simulink model "detumbling"  (R2021a)
settings: Solver=VariableStepAuto  StartTime=0.0  StopTime=3*Torb  RelTol=1e-3
values from neighbouring files (symbols this model uses):
  inc = 0    [params_detumb.m]    (also in params_nadir.m; params_roll.m)
  Torb = 2*pi*sqrt(norm(r0)^3/mu)    [params_detumb.m]    (also in params_nadir.m; params_roll.m)
libraries: sharedtransform x5, aerolibutil x2
settings Model: Creator=Laura  LastModifiedBy=Laura

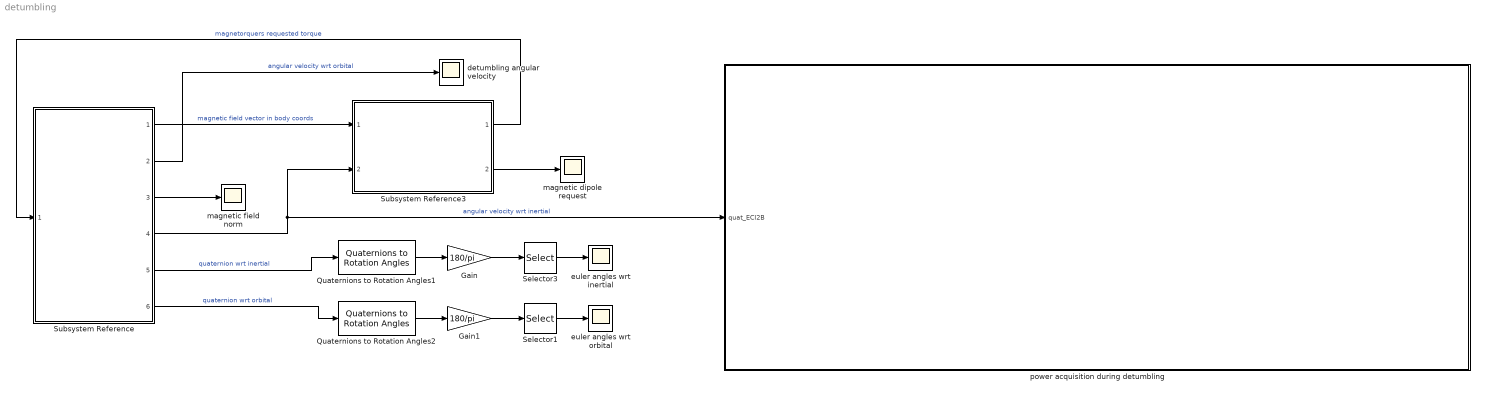
== system detumbling ==
  Gain : Gain  Gain=180/pi
  Gain1 : Gain  Gain=180/pi
  Quaternions to Rotation Angles1 : sharedtransform/Quaternions to Rotation Angles  rotationOrder=ZYX  aMode=aMode
      settings: SourceProductBaseCode=AE,PW,DR,MT,UV,VE
  Quaternions to Rotation Angles2 : sharedtransform/Quaternions to Rotation Angles  rotationOrder=ZYX  aMode=aMode
      settings: SourceProductBaseCode=AE,PW,DR,MT,UV,VE
  Selector1 : Selector  InputPortWidth=3  IndexOptions=Index vector (dialog)  Indices=[3 2 1]  OutputSizes=1
  Selector3 : Selector  InputPortWidth=3  IndexOptions=Index vector (dialog)  Indices=[3 2 1]  OutputSizes=1
  Subsystem Reference : Subsystem  ReferencedSubsystem=DKE
  Subsystem Reference3 : Subsystem  ReferencedSubsystem=BdotController
  detumbling angular velocity : Scope
  euler angles wrt inertial : Scope
  euler angles wrt orbital : Scope
  magnetic dipole request : Scope
  magnetic field norm : Scope
  power acquisition during detumbling : Subsystem
  wires:
  Quaternions to Rotation Angles1/1 -> Gain/1
  Gain/1 -> Selector3/1
  Selector3/1 -> euler angles wrt inertial/1
  Subsystem Reference/1 -> Subsystem Reference3/1  "magnetic field vector in body coords"
  Subsystem Reference/2 -> detumbling angular velocity/1  "angular velocity wrt orbital"
  Subsystem Reference3/1 -> Subsystem Reference/1  "magnetorquers requested torque"
  Quaternions to Rotation Angles2/1 -> Gain1/1
  Subsystem Reference/4 -> power acquisition during detumbling/1(quat_ECI2B), Subsystem Reference3/2  "angular velocity wrt inertial"
  Subsystem Reference/3 -> magnetic field norm/1
  Gain1/1 -> Selector1/1
  Selector1/1 -> euler angles wrt orbital/1
  Subsystem Reference/6 -> Quaternions to Rotation Angles2/1  "quaternion wrt orbital"
  Subsystem Reference/5 -> Quaternions to Rotation Angles1/1  "quaternion wrt inertial"
  Subsystem Reference3/2 -> magnetic dipole request/1

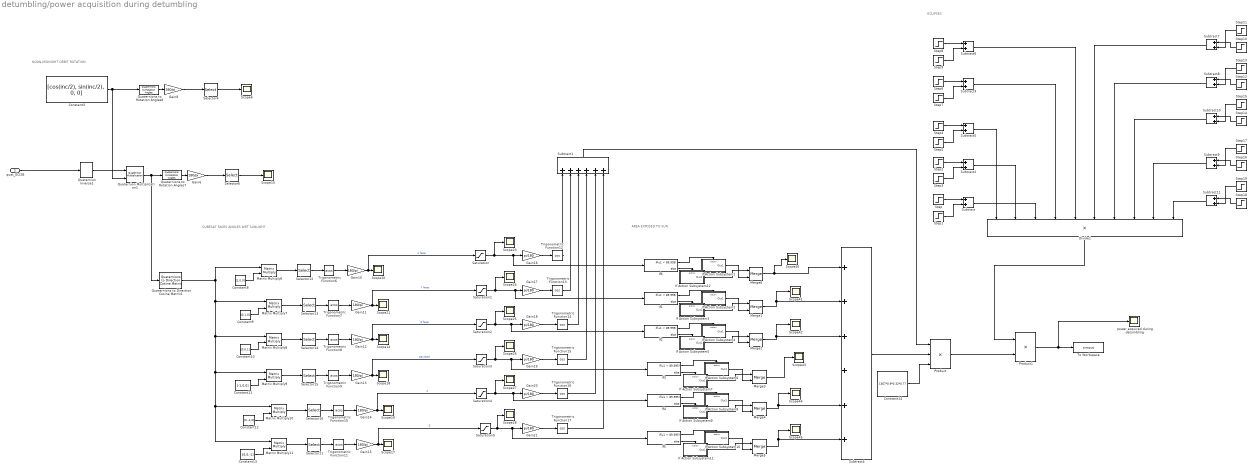
== system detumbling/power acquisition during detumbling ==
  note: AREA EXPOSED TO SUN
  note: ECLIPSES
  note: CUBESAT FACES ANGLES WRT SUNLIGHT
  note: NOON-MIDNIGHT ORBIT ROTATION
  quat_ECI2B : Inport
  Constant10 : Constant  Value=[0,0,1]
  Constant11 : Constant  Value=[-1,0,0]
  Constant12 : Constant  Value=[0,-1,0]
  Constant13 : Constant  Value=[0,0,-1]
  Constant14 : Constant  Value=1367*0.9*0.32*0.77
  Constant3 : Constant  Value=[cos(inc/2), sin(inc/2), 0, 0]
  Constant8 : Constant  Value=[1,0,0]
  Constant9 : Constant  Value=[0,1,0]
  Divide1 : Product  Inputs=**********
  Gain{6,8,10..15} (8 alike) : Gain  Gain=180/pi
  Gain{16..21} (6 alike) : Gain  Gain=pi/180
  If Action Subsystem1 : Subsystem  TreatAsAtomicUnit=on
  If Action Subsystem10 : Subsystem  TreatAsAtomicUnit=on
  If Action Subsystem11 : Subsystem  TreatAsAtomicUnit=on
  If Action Subsystem12 : Subsystem  TreatAsAtomicUnit=on
  If Action Subsystem2 : Subsystem  TreatAsAtomicUnit=on
  If Action Subsystem3 : Subsystem  TreatAsAtomicUnit=on
  If Action Subsystem4 : Subsystem  TreatAsAtomicUnit=on
  If Action Subsystem5 : Subsystem  TreatAsAtomicUnit=on
  If Action Subsystem6 : Subsystem  TreatAsAtomicUnit=on
  If Action Subsystem7 : Subsystem  TreatAsAtomicUnit=on
  If Action Subsystem8 : Subsystem  TreatAsAtomicUnit=on
  If Action Subsystem9 : Subsystem  TreatAsAtomicUnit=on
  If{1..6} (6 alike) : If  IfExpression=u1 < 89.995
  Matrix Multiply{6..11} (6 alike) : Product  Multiplication=Matrix(*)
  Merge{1..6} (6 alike) : Merge
  Product : Product  Inputs=3
  Product1 : Product
  Quaternion Inverse1 : aerolibutil/Quaternion Inverse
  Quaternion Multiplication1 : aerolibutil/Quaternion Multiplication
  Quaternions to Direction Cosine Matrix1 : sharedtransform/Quaternions to  Direction Cosine Matrix  aMode=aMode
      settings: SourceProductBaseCode=AE,PW,DR,MT,UV,VE
  Quaternions to Rotation Angles7 : sharedtransform/Quaternions to Rotation Angles  rotationOrder=ZYX  aMode=aMode
      settings: SourceProductBaseCode=AE,PW,DR,MT,UV,VE
  Quaternions to Rotation Angles8 : sharedtransform/Quaternions to Rotation Angles  rotationOrder=ZYX  aMode=aMode
      settings: SourceProductBaseCode=AE,PW,DR,MT,UV,VE
  Saturation{,1..5} (6 alike) : Saturate  UpperLimit=90.00005  LowerLimit=-90.00005
  Scope{6,10,14,17..21,23..28,40..45} (20 alike) : Scope
  Selector{11..16} (6 alike) : Selector  InputPortWidth=3  IndexOptions=Index vector (dialog)  Indices=[1]  OutputSizes=1
  Selector4 : Selector  InputPortWidth=3  IndexOptions=Index vector (dialog)  Indices=[3 2 1]  OutputSizes=1
  Selector6 : Selector  InputPortWidth=3  IndexOptions=Index vector (dialog)  Indices=[3 2 1]  OutputSizes=1
  Step : Step  Time=30.76*60  Before=1  After=0  SampleTime=0
  Step1 : Step  Time=(30.76 + 35)*60  SampleTime=0
  Step10 : Step  Time=30.76*60 + 10*Torb  Before=1  After=0  SampleTime=0
  Step11 : Step  Time=(30.76 + 35)*60 + 10*Torb  SampleTime=0
  Step12 : Step  Time=30.76*60 + 9*Torb  Before=1  After=0  SampleTime=0
  Step13 : Step  Time=(30.76 + 35)*60 + 9*Torb  SampleTime=0
  Step14 : Step  Time=30.76*60 + 8*Torb  Before=1  After=0  SampleTime=0
  Step15 : Step  Time=(30.76 + 35)*60 + 8*Torb  SampleTime=0
  Step16 : Step  Time=30.76*60 + 7*Torb  Before=1  After=0  SampleTime=0
  Step17 : Step  Time=(30.76 + 35)*60 + 7*Torb  SampleTime=0
  Step18 : Step  Time=30.76*60 + 6*Torb  Before=1  After=0  SampleTime=0
  Step19 : Step  Time=(30.76 + 35)*60 + 6*Torb  SampleTime=0
  Step2 : Step  Time=30.76*60 + Torb  Before=1  After=0  SampleTime=0
  Step3 : Step  Time=(30.76 + 35)*60 + Torb  SampleTime=0
  Step4 : Step  Time=30.76*60 + 2*Torb  Before=1  After=0  SampleTime=0
  Step5 : Step  Time=(30.76 + 35)*60 + 2*Torb  SampleTime=0
  Step6 : Step  Time=30.76*60 + 4*Torb  Before=1  After=0  SampleTime=0
  Step7 : Step  Time=(30.76 + 35)*60 + 4*Torb  SampleTime=0
  Step8 : Step  Time=30.76*60 + 5*Torb  Before=1  After=0  SampleTime=0
  Step9 : Step  Time=(30.76 + 35)*60 + 5*Torb  SampleTime=0
  Subtract{,2..3,5..11} (10 alike) : Sum
  Subtract1 : Sum  Inputs=++++++
  Subtract4 : Sum  Inputs=++++++
  To Workspace : ToWorkspace  VariableName=simout  SaveFormat=Timeseries  SampleTime=-1
  Trigonometric Function{6..11} (6 alike) : Trigonometry  Operator=acos
  Trigonometric Function{12..17} (6 alike) : Trigonometry  Operator=cos
  power acquired during detumbling : Scope
  wires:
  Subtract/1 -> Divide1/3
  Step17/1 -> Subtract9/2
  Subtract9/1 -> Divide1/9
  Gain6/1 -> Selector6/1
  Subtract8/1 -> Divide1/7
  Gain21/1 -> Trigonometric Function17/1
  Constant3/1 -> Quaternions to Rotation Angles8/1, Quaternion Multiplication1/2
  Subtract1/1 -> Product/1
  Step18/1 -> Subtract11/1
  Step7/1 -> Subtract3/2
  Step10/1 -> Subtract7/1
  Selector11/1 -> Trigonometric Function11/1
  If Action Subsystem11/1(Out1) -> Merge5/1
  Saturation1/1 -> If1/1, Gain17/1, Scope24/1
  Step15/1 -> Subtract10/2
  Step19/1 -> Subtract11/2
  Step13/1 -> Subtract8/2
  Step6/1 -> Subtract3/1
  Gain12/1 -> Saturation2/1, Scope14/1  "Z face"
  Trigonometric Function12/1 -> Subtract1/1
  Step11/1 -> Subtract7/2
  Step8/1 -> Subtract6/1
  If Action Subsystem2/1(Out1) -> Merge1/2
  Merge2/1 -> Scope42/1, Subtract4/3
  Step16/1 -> Subtract9/1
  Trigonometric Function8/1 -> Gain12/1
  Matrix Multiply10/1 -> Selector16/1
  Divide1/1 -> Product1/1
  Selector14/1 -> Trigonometric Function8/1
  Step1/1 -> Subtract/2
  Step/1 -> Subtract/1
  Step3/1 -> Subtract2/2
  Step2/1 -> Subtract2/1
  Gain11/1 -> Saturation1/1, Scope21/1  "Y face"
  If4/1 -> If Action Subsystem8/Action
  Gain18/1 -> Trigonometric Function14/1
  If Action Subsystem8/1(Out1) -> Merge4/2
  Matrix Multiply9/1 -> Selector15/1
  Selector16/1 -> Trigonometric Function10/1
  Saturation5/1 -> If5/1, Gain21/1, Scope28/1
  If Action Subsystem9/1(Out1) -> Merge4/1
  Subtract2/1 -> Divide1/2
  Quaternions to Direction Cosine Matrix1/1 -> Matrix Multiply6/1, Matrix Multiply8/1, Matrix Multiply9/1, Matrix Multiply10/1, Matrix Multiply11/1, Matrix Multiply7/1
  If1/2 -> If Action Subsystem3/Action
  Constant12/1 -> Matrix Multiply10/2
  If5/2 -> If Action Subsystem11/Action
  If Action Subsystem1/1(Out1) -> Merge6/2
  Trigonometric Function9/1 -> Gain13/1
  Constant8/1 -> Matrix Multiply6/2
  If3/1 -> If Action Subsystem6/Action
  Merge4/1 -> Scope44/1, Subtract4/5
  Constant9/1 -> Matrix Multiply7/2
  Constant10/1 -> Matrix Multiply8/2
  Matrix Multiply7/1 -> Selector13/1
  If Action Subsystem10/1(Out1) -> Merge5/2
  If5/1 -> If Action Subsystem10/Action
  Selector12/1 -> Trigonometric Function6/1
  Saturation/1 -> If6/1, Gain16/1, Scope23/1
  If2/1 -> If Action Subsystem4/Action
  Step5/1 -> Subtract5/2
  Selector15/1 -> Trigonometric Function9/1
  Gain13/1 -> Saturation3/1, Scope18/1  "payload"
  If Action Subsystem7/1(Out1) -> Merge3/1
  Product1/1 -> power acquired during detumbling/1, To Workspace/1
  Trigonometric Function16/1 -> Subtract1/5
  Trigonometric Function7/1 -> Gain11/1
  If Action Subsystem4/1(Out1) -> Merge2/2
  If Action Subsystem5/1(Out1) -> Merge2/1
  Step14/1 -> Subtract10/1
  Merge3/1 -> Scope43/1
  Trigonometric Function14/1 -> Subtract1/3
  Gain10/1 -> Saturation/1, Scope20/1  "X face"
  Constant13/1 -> Matrix Multiply11/2
  Merge5/1 -> Scope45/1, Subtract4/6
  Trigonometric Function17/1 -> Subtract1/6
  Product/1 -> Product1/2
  If6/2 -> If Action Subsystem12/Action
  Subtract4/1 -> Product/2
  Trigonometric Function13/1 -> Subtract1/2
  Gain19/1 -> Trigonometric Function15/1
  Trigonometric Function15/1 -> Subtract1/4
  Saturation3/1 -> If3/1, Gain19/1, Scope26/1
  Gain17/1 -> Trigonometric Function13/1
  Gain14/1 -> Saturation4/1, Scope19/1  "-Y"
  If6/1 -> If Action Subsystem1/Action
  Matrix Multiply8/1 -> Selector14/1
  Step4/1 -> Subtract5/1
  Constant14/1 -> Product/3
  Trigonometric Function10/1 -> Gain14/1
  If4/2 -> If Action Subsystem9/Action
  Matrix Multiply11/1 -> Selector11/1
  Selector13/1 -> Trigonometric Function7/1
  If3/2 -> If Action Subsystem7/Action
  Quaternions to Rotation Angles7/1 -> Gain6/1
  Gain16/1 -> Trigonometric Function12/1
  Subtract5/1 -> Divide1/1
  Quaternions to Rotation Angles8/1 -> Gain8/1
  Selector4/1 -> Scope6/1
  Gain20/1 -> Trigonometric Function16/1
  Constant11/1 -> Matrix Multiply9/2
  Subtract11/1 -> Divide1/10
  If1/1 -> If Action Subsystem2/Action
  Subtract6/1 -> Divide1/5
  Gain15/1 -> Saturation5/1, Scope17/1  "-Z"
  If Action Subsystem6/1(Out1) -> Merge3/2
  Saturation2/1 -> If2/1, Gain18/1, Scope25/1
  Step12/1 -> Subtract8/1
  Merge1/1 -> Scope41/1, Subtract4/2
  Subtract10/1 -> Divide1/8
  Gain8/1 -> Selector4/1
  Subtract3/1 -> Divide1/4
  Trigonometric Function6/1 -> Gain10/1
  quat_ECI2B/1 -> Quaternion Inverse1/1
  If2/2 -> If Action Subsystem5/Action
  Step9/1 -> Subtract6/2
  If Action Subsystem12/1(Out1) -> Merge6/1
  Saturation4/1 -> Gain20/1, If4/1, Scope27/1
  Matrix Multiply6/1 -> Selector12/1
  Subtract7/1 -> Divide1/6
  Quaternion Inverse1/1 -> Quaternion Multiplication1/1
  Selector6/1 -> Scope10/1
  If Action Subsystem3/1(Out1) -> Merge1/1
  Quaternion Multiplication1/1 -> Quaternions to Direction Cosine Matrix1/1, Quaternions to Rotation Angles7/1
  Trigonometric Function11/1 -> Gain15/1
  Merge6/1 -> Subtract4/1, Scope40/1

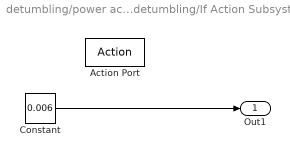
== system detumbling/power acquisition during detumbling/If Action Subsystem1 ==
  Action Port : ActionPort  ActionPortLabel=if(u1 < 89.995)
  Constant : Constant  Value=0.006
  Out1 : Outport
  wires:
  Constant/1 -> Out1/1

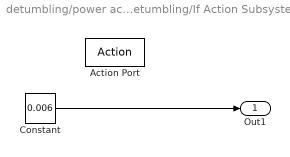
== system detumbling/power acquisition during detumbling/If Action Subsystem10 ==
  Action Port : ActionPort  ActionPortLabel=if(u1 < 89.995)
  Constant : Constant  Value=0.006
  Out1 : Outport
  wires:
  Constant/1 -> Out1/1

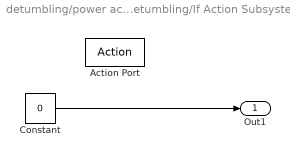
== system detumbling/power acquisition during detumbling/If Action Subsystem11 ==
  Action Port : ActionPort  ActionPortLabel=else
  Constant : Constant  Value=0
  Out1 : Outport
  wires:
  Constant/1 -> Out1/1

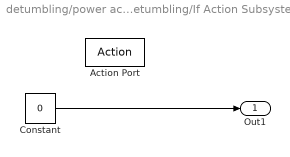
== system detumbling/power acquisition during detumbling/If Action Subsystem12 ==
  Action Port : ActionPort  ActionPortLabel=else
  Constant : Constant  Value=0
  Out1 : Outport
  wires:
  Constant/1 -> Out1/1

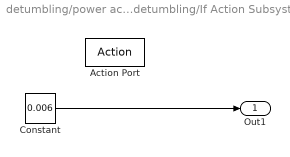
== system detumbling/power acquisition during detumbling/If Action Subsystem2 ==
  Action Port : ActionPort  ActionPortLabel=if(u1 < 89.995)
  Constant : Constant  Value=0.006
  Out1 : Outport
  wires:
  Constant/1 -> Out1/1

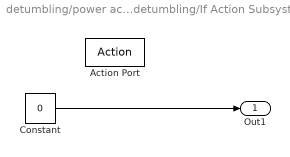
== system detumbling/power acquisition during detumbling/If Action Subsystem3 ==
  Action Port : ActionPort  ActionPortLabel=else
  Constant : Constant  Value=0
  Out1 : Outport
  wires:
  Constant/1 -> Out1/1

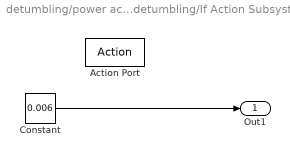
== system detumbling/power acquisition during detumbling/If Action Subsystem4 ==
  Action Port : ActionPort  ActionPortLabel=if(u1 < 89.995)
  Constant : Constant  Value=0.006
  Out1 : Outport
  wires:
  Constant/1 -> Out1/1

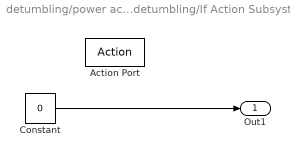
== system detumbling/power acquisition during detumbling/If Action Subsystem5 ==
  Action Port : ActionPort  ActionPortLabel=else
  Constant : Constant  Value=0
  Out1 : Outport
  wires:
  Constant/1 -> Out1/1

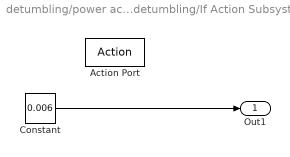
== system detumbling/power acquisition during detumbling/If Action Subsystem6 ==
  Action Port : ActionPort  ActionPortLabel=if(u1 < 89.995)
  Constant : Constant  Value=0.006
  Out1 : Outport
  wires:
  Constant/1 -> Out1/1

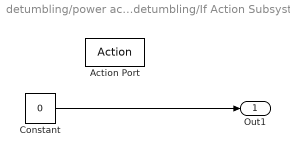
== system detumbling/power acquisition during detumbling/If Action Subsystem7 ==
  Action Port : ActionPort  ActionPortLabel=else
  Constant : Constant  Value=0
  Out1 : Outport
  wires:
  Constant/1 -> Out1/1

== system detumbling/power acquisition during detumbling/If Action Subsystem8 ==
  Action Port : ActionPort  ActionPortLabel=if(u1 < 89.995)
  Constant : Constant  Value=0.003
  Out1 : Outport
  wires:
  Constant/1 -> Out1/1

== system detumbling/power acquisition during detumbling/If Action Subsystem9 ==
  Action Port : ActionPort  ActionPortLabel=else
  Constant : Constant  Value=0
  Out1 : Outport
  wires:
  Constant/1 -> Out1/1
